simulink library "Compressor_Defaults"  (R2019b)
settings: Solver=ode45  StartTime=0.0  StopTime=10.0  RelTol=1e-3  EnableMultiTasking=on
undefined symbols (not defined in the file): kg, s
libraries: simulink x2
settings Model: Creator=mbrauer  LastModifiedBy=bhisma
settings DataIOCC: LimitDataPoints=on  SaveFormat=Array  SignalLoggingSaveFormat=ModelDataLogs  ReturnWorkspaceOutputs=off
settings OptimizationCC: LifeSpan=inf
settings DebuggingCC: SolverPrmCheckMsg=warning  MultiTaskDSMMsg=warning  MultiTaskCondExecSysMsg=none  SFUnexpectedBacktrackingDiag=warning  SFNoUnconditionalDefaultTransitionDiag=warning  SFExecutionAtInitializationDiag=none  ArithmeticOperatorsInVariantConditions=warning
settings HardwareCC: ProdBitPerPointer=32  ProdBitPerSizeT=32  ProdBitPerPtrDiffT=32  ProdLargestAtomicFloat=None  ProdIntDivRoundTo=Undefined  ProdEndianess=Unspecified  ProdWordSize=32  ProdHWDeviceType=32-bit Generic
settings ModelReferenceCC: PropagateSignalLabelsOutOfModel=off
settings SFSimCC: SimUseLocalCustomCode=off  CustomCodeUndefinedFunction=UseInterfaceOnly
settings RTWCC: RTWUseLocalCustomCode=off
settings CodeAppCC: StateflowObjectComments=on
settings GRTTargetCC: TargetLangStandard=C89/C90 (ANSI)  GeneratePreprocessorConditionals=Disable all
settings ConfigComp: CovMetricSettings=dw  CovHtmlReporting=on  CovSaveCumulativeToWorkspaceVar=on  CovSaveSingleToWorkspaceVar=on  CovExternalEMLEnable=off

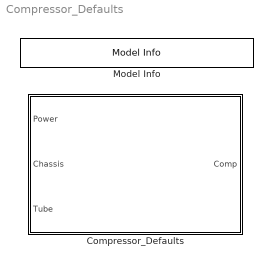
== system Compressor_Defaults ==
  Compressor_Defaults : Subsystem  VariantControl=VAR_Compressor_Defaults
  Model Info : simulink/Model-Wide Utilities/Model Info  Frame=on  DisplayStringWithTags=Copyright 2013-2014 The MathWorks, Inc.  HorizontalTextAlignment=Center  LeftAlignmentValue=0.5

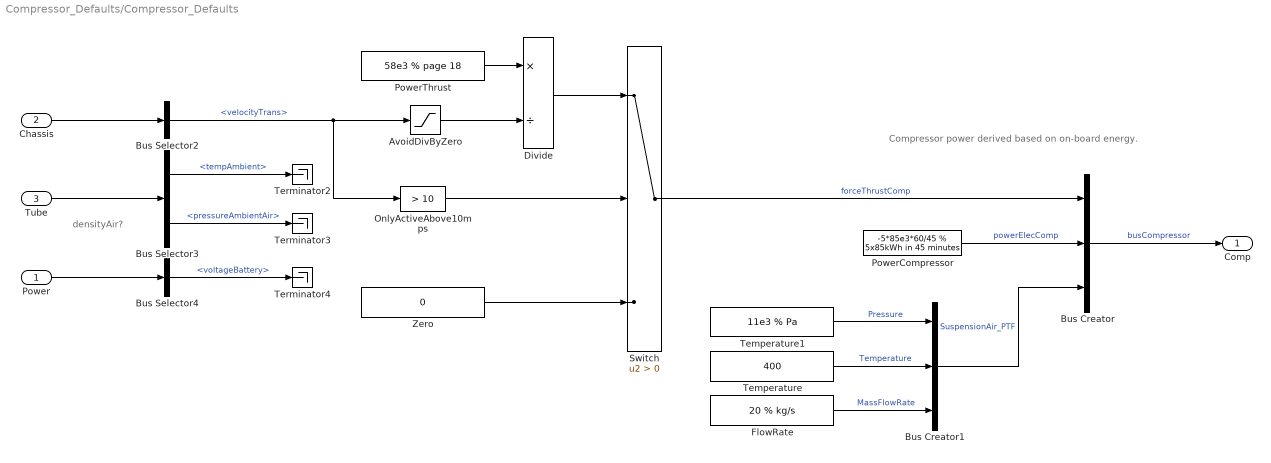
== system Compressor_Defaults/Compressor_Defaults ==
  note: Compressor power derived based on on-board energy.
  note: densityAir?
  Power : Inport
  Chassis : Inport  Port=2
  Tube : Inport  Port=3
  AvoidDivByZero : Saturate  UpperLimit=inf  LowerLimit=1
      settings: AttributesFormatString=|
      | UL = %<UpperLimit>
      | LL = %<LowerLimit>
  Bus Creator : BusCreator  Inputs=3  NonVirtualBus=on
  Bus Creator1 : BusCreator  Inputs=3
  Bus Selector2 : BusSelector  OutputSignals=velocityTrans
  Bus Selector3 : BusSelector  OutputSignals=tempAmbient,pressureAmbientAir
  Bus Selector4 : BusSelector  OutputSignals=voltageBattery
  Divide : Product  Inputs=*/
  FlowRate : Constant  Value=20 % kg/s
  OnlyActiveAbove10mps : simulink/Logic and Bit Operations/Compare To Constant  relop=>  const=10  OutDataTypeStr=boolean
  PowerCompressor : Constant  Value=-5*85e3*60/45 % 5x85kWh in 45 minutes
  PowerThrust : Constant  Value=58e3 % page 18
  Switch : Switch  Criteria=u2 > Threshold
  Temperature : Constant  Value=400
  Temperature1 : Constant  Value=11e3 % Pa
  Terminator2 : Terminator
  Terminator3 : Terminator
  Terminator4 : Terminator
  Zero : Constant  Value=0
  Comp : Outport
  wires:
  FlowRate/1 -> Bus Creator1/3  "MassFlowRate"
  Temperature/1 -> Bus Creator1/2  "Temperature"
  Temperature1/1 -> Bus Creator1/1  "Pressure"
  Bus Creator1/1 -> Bus Creator/3  "SuspensionAir_PTF"
  Bus Creator/1 -> Comp/1  "busCompressor"
  Switch/1 -> Bus Creator/1  "forceThrustComp"
  PowerCompressor/1 -> Bus Creator/2  "powerElecComp"
  Chassis/1 -> Bus Selector2/1
  Tube/1 -> Bus Selector3/1
  Bus Selector2/1 -> OnlyActiveAbove10mps/1, AvoidDivByZero/1  "<velocityTrans>"
  Bus Selector3/1 -> Terminator2/1  "<tempAmbient>"
  Bus Selector3/2 -> Terminator3/1  "<pressureAmbientAir>"
  Power/1 -> Bus Selector4/1
  Bus Selector4/1 -> Terminator4/1  "<voltageBattery>"
  PowerThrust/1 -> Divide/1
  Divide/1 -> Switch/1
  OnlyActiveAbove10mps/1 -> Switch/2
  Zero/1 -> Switch/3
  AvoidDivByZero/1 -> Divide/2
